simulink model "modell"  (R2023a)
settings: Solver=VariableStepAuto  StartTime=0.0  StopTime=40.0  RelTol=1e-3
InitFcn:
  | %rendszermátrixok
  | A = ...
  |     [-0.313 57.7 0;
  |     -0.0139 -0.426 0;
  |     0 56.7 0];
  | B = ...
  |     [0.232;
  |     0.0203;
  |     0];
  | C = [0 0 1];
  | D = 0;
  | 
  | %visszacsatoló erősítést
  | K = [-0.6435 169.6950 7.0711];
  | 
  | %előerősítő értéke
  | N = 7.0711;
  | 
  | %módosított rendszermátrix
  | B_mod = ...
  |     [0.232*1.4;
  |     0.0203*0.6;
  |     0];
settings Model: Creator=vadav  LastModifiedBy=vadav

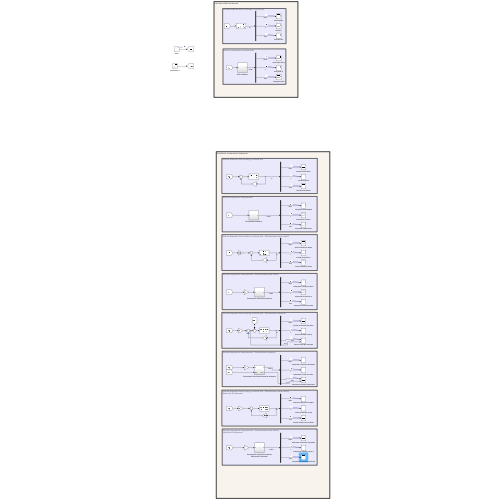
[thumbnail: Simulink's stored preview of the top-level diagram]
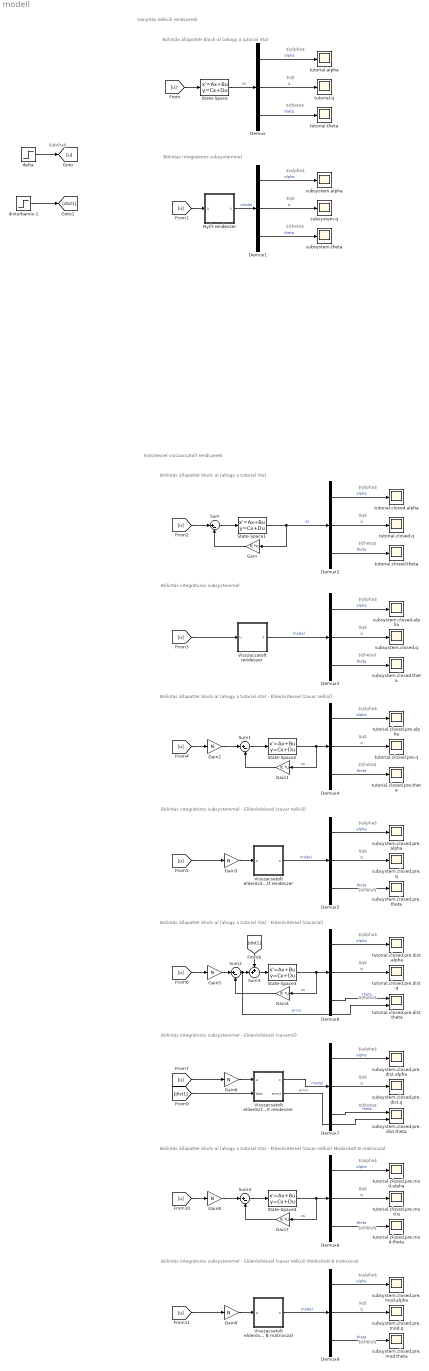
== system modell ==
  note: Erősítéssel visszacsatolt rendszerek
  note: Bólintás integrátoros subsystemmel
  note: Bólintás állapottér block-al (ahogy a tutorial írta)
  note: $\alpha$
  note: $q$
  note: $\theta$
  note: $\delta$
  note: $\alpha$
  note: $q$
  note: $\theta$
  note: Bólintás állapottér block-al (ahogy a tutorial írta)
  note: $\alpha$
  note: $q$
  note: $\theta$
  note: $\theta$
  note: $q$
  note: Bólintás integrátoros subsystemmel
  note: $\alpha$
  note: Irányítás nélküli rendszerek
  note: $\theta$
  note: $q$
  note: $q$
  note: $\alpha$
  note: $\theta$
  note: Bólintás integrátoros subsystemmel - Előerősítéssel (zavar nélkül)
  note: $\alpha$
  note: Bólintás állapottér block-al (ahogy a tutorial írta) - Előerősítéssel (zavar nélkül)
  note: $\theta$
  note: $q$
  note: Bólintás integrátoros subsystemmel - Előerősítéssel (zavarral)
  note: Bólintás állapottér block-al (ahogy a tutorial írta) - Előerősítéssel (zavarral)
  note: $q$
  note: $\alpha$
  note: $\alpha$
  note: $\theta$
  note: $\theta$
  note: $q$
  note: Bólintás integrátoros subsystemmel - Előerősítéssel (zavar nélkül)
      | Módosított B mátrixszal
  note: Bólintás állapottér block-al (ahogy a tutorial írta) - Előerősítéssel (zavar nélkül)
      | Módosított B mátrixszal
  note: $q$
  note: $\alpha$
  note: $\alpha$
  note: $\theta$
  Demux{,1..9} (10 alike) : Demux  Outputs=3
  Gain{,1,4,7} (4 alike) : Gain  Gain=K  Multiplication=Matrix(K*u)
  Gain{2..3,5..6,8..9} (6 alike) : Gain  Gain=N
  Nyílt rendeszer : Subsystem
  State-Space{,1..3} (4 alike) : StateSpace  A=A  B=B  C=eye(3)  D=[0;0;0]  InitialCondition=0  ContinuousStateAttributes={'Allasszog', 'Bolintas_valtozasa', 'Bolintas'}
  State-Space4 : StateSpace  A=A  B=B_mod  C=eye(3)  D=[0;0;0]  InitialCondition=0  ContinuousStateAttributes={'Allasszog', 'Bolintas_valtozasa', 'Bolintas'}
  Sum{,1..2,4} (4 alike) : Sum  Inputs=|+-
  Sum3 : Sum  Inputs=++|
  Visszacsatolt előerősített megzavart rendeszer : Subsystem
  Visszacsatolt előerősített rendeszer : Subsystem
  Visszacsatolt előerősített rendeszer Módosított B mátrixszal : Subsystem
  Visszacsatolt rendeszer : Subsystem
  delta : Step  Time=0  After=0.2  SampleTime=0
  disturbance-1 : Step  Time=3  After=0.2  SampleTime=0
  subsystem.alpha : Scope
  subsystem.closed.alpha : Scope
  subsystem.closed.pre.alpha : Scope
  subsystem.closed.pre.dist.alpha : Scope
  subsystem.closed.pre.dist.q : Scope
  subsystem.closed.pre.dist.theta : Scope  NumInputPorts=2
  subsystem.closed.pre.mod.alpha : Scope
  subsystem.closed.pre.mod.q : Scope
  subsystem.closed.pre.mod.theta : Scope
  subsystem.closed.pre.q : Scope
  subsystem.closed.pre.theta : Scope
  subsystem.closed.q : Scope
  subsystem.closed.theta : Scope
  subsystem.q : Scope
  subsystem.theta : Scope
  tutorial.alpha : Scope
  tutorial.closed.alpha : Scope
  tutorial.closed.pre.alpha : Scope
  tutorial.closed.pre.dist.alpha : Scope
  tutorial.closed.pre.dist.q : Scope
  tutorial.closed.pre.dist.theta : Scope  NumInputPorts=2
  tutorial.closed.pre.mod.alpha : Scope
  tutorial.closed.pre.mod.q : Scope
  tutorial.closed.pre.mod.theta : Scope
  tutorial.closed.pre.q : Scope
  tutorial.closed.pre.theta : Scope
  tutorial.closed.q : Scope
  tutorial.closed.theta : Scope
  tutorial.q : Scope
  tutorial.theta : Scope
  wires:
  Demux/3 -> tutorial.theta/1  "theta"
  Demux/1 -> tutorial.alpha/1  "alpha"
  Demux/2 -> tutorial.q/1  "q"
  State-Space/1 -> Demux/1  "ss"
  [u] -> State-Space/1
  [u] -> Nyílt rendeszer/1(u)
  Nyílt rendeszer/1(x) -> Demux1/1  "model"
  Demux1/2 -> subsystem.q/1  "q"
  Demux1/1 -> subsystem.alpha/1  "alpha"
  Demux1/3 -> subsystem.theta/1  "theta"
  State-Space1/1 -> Gain/1, Demux2/1  "ss"
  Demux2/2 -> tutorial.closed.q/1  "q"
  Demux2/1 -> tutorial.closed.alpha/1  "alpha"
  Demux2/3 -> tutorial.closed.theta/1  "theta"
  [u] -> Sum/1
  Sum/1 -> State-Space1/1
  Gain/1 -> Sum/2
  Demux3/1 -> subsystem.closed.alpha/1  "alpha"
  Demux3/3 -> subsystem.closed.theta/1  "theta"
  Demux3/2 -> subsystem.closed.q/1  "q"
  Visszacsatolt rendeszer/1(x) -> Demux3/1  "model"
  [u] -> Visszacsatolt rendeszer/1(u)
  Demux5/2 -> subsystem.closed.pre.q/1  "q"
  Visszacsatolt előerősített rendeszer/1(x) -> Demux5/1  "model"
  Demux5/1 -> subsystem.closed.pre.alpha/1  "alpha"
  Demux4/3 -> tutorial.closed.pre.theta/1  "theta"
  Demux5/3 -> subsystem.closed.pre.theta/1  "theta"
  Demux4/2 -> tutorial.closed.pre.q/1  "q"
  State-Space2/1 -> Gain1/1, Demux4/1  "ss"
  Demux4/1 -> tutorial.closed.pre.alpha/1  "alpha"
  Sum1/1 -> State-Space2/1
  Gain1/1 -> Sum1/2
  [u] -> Gain2/1
  Gain2/1 -> Sum1/1
  [u] -> Gain3/1
  Gain3/1 -> Visszacsatolt előerősített rendeszer/1(u)
  Gain4/1 -> Sum2/2
  Demux6/2 -> tutorial.closed.pre.dist.q/1  "q"
  Demux6/3 -> tutorial.closed.pre.dist.theta/1  "theta"
  Demux6/1 -> tutorial.closed.pre.dist.alpha/1  "alpha"
  State-Space3/1 -> Gain4/1, Demux6/1  "ss"
  Demux7/1 -> subsystem.closed.pre.dist.alpha/1  "alpha"
  Demux7/2 -> subsystem.closed.pre.dist.q/1  "q"
  [u] -> Gain6/1
  Demux7/3 -> subsystem.closed.pre.dist.theta/1  "theta"
  [u] -> Gain5/1
  Gain6/1 -> Visszacsatolt előerősített megzavart rendeszer/1(u)
  Visszacsatolt előerősített megzavart rendeszer/1(x) -> Demux7/1  "model"
  Gain5/1 -> Sum2/1
  disturbance-1/1 -> [dist1]
  Sum2/1 -> tutorial.closed.pre.dist.theta/2, Sum3/2  "error"
  Sum3/1 -> State-Space3/1
  [dist1] -> Sum3/1
  delta/1 -> [u]
  [dist1] -> Visszacsatolt előerősített megzavart rendeszer/2(dist)
  Visszacsatolt előerősített megzavart rendeszer/2(error) -> subsystem.closed.pre.dist.theta/2  "error"
  Sum4/1 -> State-Space4/1
  Gain7/1 -> Sum4/2
  Demux8/2 -> tutorial.closed.pre.mod.q/1  "q"
  Demux8/3 -> tutorial.closed.pre.mod.theta/1  "theta"
  Demux8/1 -> tutorial.closed.pre.mod.alpha/1  "alpha"
  State-Space4/1 -> Gain7/1, Demux8/1  "ss"
  Demux9/1 -> subsystem.closed.pre.mod.alpha/1  "alpha"
  Demux9/2 -> subsystem.closed.pre.mod.q/1  "q"
  [u] -> Gain9/1
  Demux9/3 -> subsystem.closed.pre.mod.theta/1  "theta"
  [u] -> Gain8/1
  Gain9/1 -> Visszacsatolt előerősített rendeszer Módosított B mátrixszal/1(u)
  Visszacsatolt előerősített rendeszer Módosított B mátrixszal/1(x) -> Demux9/1  "model"
  Gain8/1 -> Sum4/1

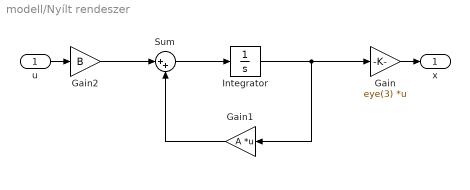
== system modell/Nyílt rendeszer ==
  u : Inport
  Gain : Gain  Gain=eye(3)  Multiplication=Matrix(K*u)
  Gain1 : Gain  Gain=A  Multiplication=Matrix(K*u)
  Gain2 : Gain  Gain=B
  Integrator : Integrator  ContinuousStateAttributes={'Allasszog', 'Bolintas_valtozasa', 'Bolintas'}
  Sum : Sum  Inputs=|++
  x : Outport
  wires:
  Integrator/1 -> Gain1/1, Gain/1
  Gain2/1 -> Sum/1
  Gain/1 -> x/1
  Sum/1 -> Integrator/1
  u/1 -> Gain2/1
  Gain1/1 -> Sum/2

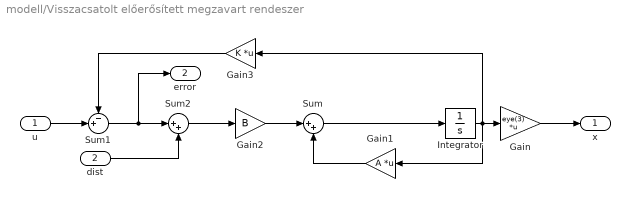
== system modell/Visszacsatolt előerősített megzavart rendeszer ==
  u : Inport
  dist : Inport  Port=2
  Gain : Gain  Gain=eye(3)  Multiplication=Matrix(K*u)
  Gain1 : Gain  Gain=A  Multiplication=Matrix(K*u)
  Gain2 : Gain  Gain=B
  Gain3 : Gain  Gain=K  Multiplication=Matrix(K*u)
  Integrator : Integrator  ContinuousStateAttributes={'Allasszog', 'Bolintas_valtozasa', 'Bolintas'}
  Sum : Sum  Inputs=|++
  Sum1 : Sum  Inputs=-+|
  Sum2 : Sum  Inputs=|++
  x : Outport
  error : Outport  Port=2
  wires:
  Gain1/1 -> Sum/2
  Gain3/1 -> Sum1/1
  Sum1/1 -> error/1, Sum2/1
  u/1 -> Sum1/2
  dist/1 -> Sum2/2
  Sum2/1 -> Gain2/1
  Gain2/1 -> Sum/1
  Sum/1 -> Integrator/1
  Integrator/1 -> Gain1/1, Gain3/1, Gain/1
  Gain/1 -> x/1

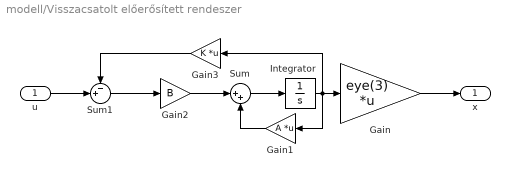
== system modell/Visszacsatolt előerősített rendeszer ==
  u : Inport
  Gain : Gain  Gain=eye(3)  Multiplication=Matrix(K*u)
  Gain1 : Gain  Gain=A  Multiplication=Matrix(K*u)
  Gain2 : Gain  Gain=B
  Gain3 : Gain  Gain=K  Multiplication=Matrix(K*u)
  Integrator : Integrator  ContinuousStateAttributes={'Allasszog', 'Bolintas_valtozasa', 'Bolintas'}
  Sum : Sum  Inputs=|++
  Sum1 : Sum  Inputs=-+|
  x : Outport
  wires:
  Integrator/1 -> Gain3/1, Gain1/1, Gain/1
  Gain1/1 -> Sum/2
  u/1 -> Sum1/2
  Sum/1 -> Integrator/1
  Sum1/1 -> Gain2/1
  Gain/1 -> x/1
  Gain3/1 -> Sum1/1
  Gain2/1 -> Sum/1

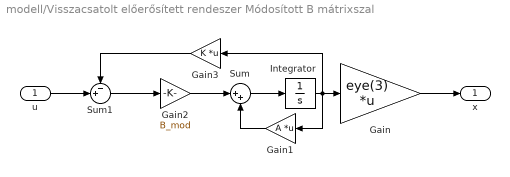
== system modell/Visszacsatolt előerősített rendeszer Módosított B mátrixszal ==
  u : Inport
  Gain : Gain  Gain=eye(3)  Multiplication=Matrix(K*u)
  Gain1 : Gain  Gain=A  Multiplication=Matrix(K*u)
  Gain2 : Gain  Gain=B_mod
  Gain3 : Gain  Gain=K  Multiplication=Matrix(K*u)
  Integrator : Integrator  ContinuousStateAttributes={'Allasszog', 'Bolintas_valtozasa', 'Bolintas'}
  Sum : Sum  Inputs=|++
  Sum1 : Sum  Inputs=-+|
  x : Outport
  wires:
  Integrator/1 -> Gain3/1, Gain1/1, Gain/1
  Gain1/1 -> Sum/2
  u/1 -> Sum1/2
  Sum/1 -> Integrator/1
  Sum1/1 -> Gain2/1
  Gain/1 -> x/1
  Gain3/1 -> Sum1/1
  Gain2/1 -> Sum/1

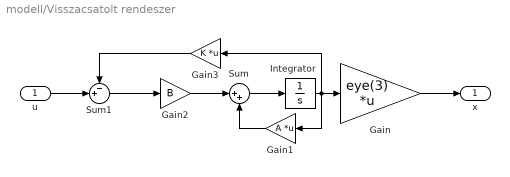
== system modell/Visszacsatolt rendeszer ==
  u : Inport
  Gain : Gain  Gain=eye(3)  Multiplication=Matrix(K*u)
  Gain1 : Gain  Gain=A  Multiplication=Matrix(K*u)
  Gain2 : Gain  Gain=B
  Gain3 : Gain  Gain=K  Multiplication=Matrix(K*u)
  Integrator : Integrator  ContinuousStateAttributes={'Allasszog', 'Bolintas_valtozasa', 'Bolintas'}
  Sum : Sum  Inputs=|++
  Sum1 : Sum  Inputs=-+|
  x : Outport
  wires:
  Integrator/1 -> Gain3/1, Gain1/1, Gain/1
  Gain1/1 -> Sum/2
  u/1 -> Sum1/2
  Sum/1 -> Integrator/1
  Sum1/1 -> Gain2/1
  Gain/1 -> x/1
  Gain3/1 -> Sum1/1
  Gain2/1 -> Sum/1
